simulink model "RflysimIndoorController_r2018b"  (R2018b)
settings: Solver=ode4  StartTime=0.0  StopTime=inf  FixedStep=ts  MaxStep=0.6  RelTol=1e-3
values from neighbouring files (symbols this model uses):
  l_v = 5    [RflyMain.m]    (also in RflyMain_N12_V6.m; RflyMain_N6_V3.m; RflyMain_N6_V4.m; RflyMain_V2.m)
  p_left_encircle = zeros(length(p_radius(:,1)),2)    [RflyMain.m]
  p_radius = [curve_x;curve_y]'    [RflyMain.m]
  p_right_encircle = zeros(length(p_radius(:,1)),2)    [RflyMain.m]
  p_target = [200,10]    [RflyMain.m]    (also in RflyMain_N12_V6.m; RflyMain_N6_V3.m; RflyMain_N6_V4.m; RflyMain_V2.m)
  ra = 0.6    [RflyMain.m]    (also in RflyMain_N12_V6.m; RflyMain_N6_V3.m; RflyMain_N6_V4.m; RflyMain_V2.m)
  rs = 0.25    [RflyMain.m]    (also in RflyMain_N12_V6.m; RflyMain_N6_V3.m; RflyMain_N6_V4.m; RflyMain_V2.m)
  tunnel_left = [90,20;147,14]    [RflyMain.m]
  tunnel_right = [90,1;147,7]    [RflyMain.m]
  v_max = 2    [RflyMain.m]    (also in RflyMain_N12_V6.m = 3; RflyMain_N6_V3.m = 3; RflyMain_N6_V4.m = 3; RflyMain_V2.m = 3)
undefined symbols (not defined in the file or in its folder): Twist
libraries: robotlib x7
settings Model: Creator=51078  LastModifiedBy=root
settings SFSimCC: SimUseLocalCustomCode=off
settings RTWCC: RTWUseLocalCustomCode=off
settings CodeAppCC: StateflowObjectComments=on

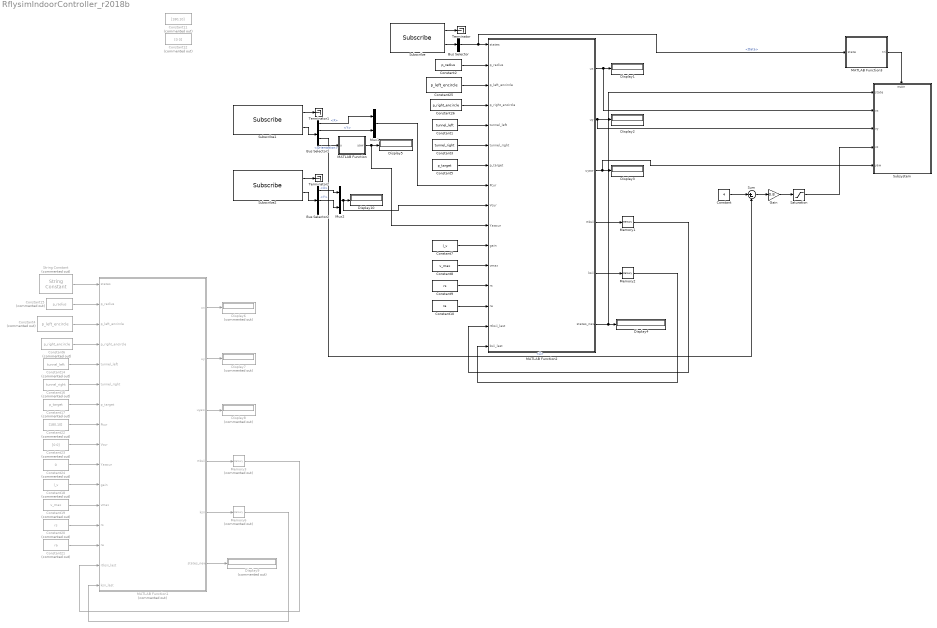
== system RflysimIndoorController_r2018b ==
  Bus Selector : BusSelector  OutputSignals=Data
  Bus Selector1 : BusSelector  OutputSignals=Pose.Position.X,Pose.Position.Y,Pose.Position.Z,Pose.Orientation
  Bus Selector2 : BusSelector  OutputSignals=Twist.Linear.X,Twist.Linear.Y,Twist.Linear.Z
  Constant : Constant  Value=4
  Constant1 : Constant  Value=tunnel_left
  Constant10 : Constant  Value=ra
  Constant11 : Constant  Commented=on  Value=[180,10]
  Constant12 : Constant  Commented=on  Value=[0 0]
  Constant14 : Constant  Commented=on  Value=tunnel_left
  Constant15 : Constant  Commented=on  Value=p_radius
  Constant16 : Constant  Commented=on  Value=tunnel_right
  Constant17 : Constant  Commented=on  Value=p_target
  Constant18 : Constant  Commented=on  Value=l_v
  Constant19 : Constant  Commented=on  Value=v_max
  Constant2 : Constant  Value=p_radius
  Constant20 : Constant  Commented=on  Value=rs
  Constant21 : Constant  Commented=on  Value=ra
  Constant22 : Constant  Commented=on  Value=[180,10]
  Constant23 : Constant  Commented=on  Value=[0 0]
  Constant24 : Constant  Commented=on  Value=0
  Constant25 : Constant  Value=p_left_encircle
  Constant26 : Constant  Value=p_right_encircle
  Constant3 : Constant  Value=tunnel_right
  Constant4 : Constant  Commented=on  Value=p_left_encircle
  Constant5 : Constant  Value=p_target
  Constant6 : Constant  Commented=on  Value=p_right_encircle
  Constant7 : Constant  Value=l_v
  Constant8 : Constant  Value=v_max
  Constant9 : Constant  Value=rs
  Display{1..5,10} (6 alike) : Display
  Display{6..9} (4 alike) : Display  Commented=on
  Gain : Gain  Gain=0.8
  MATLAB Function : MATLAB Function  TreatAsAtomicUnit=on
  MATLAB Function1 : MATLAB Function  Commented=on  TreatAsAtomicUnit=on
  MATLAB Function2 : MATLAB Function  TreatAsAtomicUnit=on
  MATLAB Function3 : MATLAB Function  TreatAsAtomicUnit=on
  Memory1 : Memory
  Memory2 : Memory
  Memory3 : Memory  Commented=on
  Memory6 : Memory  Commented=on
  Mux1 : Mux  Inputs=2
  Mux2 : Mux  Inputs=2
  Saturation : Saturate  UpperLimit=2  LowerLimit=-2
  String Constant : StringConstant  Commented=on  String="\"task_pass_through\""
  Subscribe : robotlib/Subscribe  topicSource=Select from ROS network  topic=/drone_1/state  messageType=std_msgs/UInt64  sampleTime=-1  messageQueueLength=1
  Subscribe1 : robotlib/Subscribe  topicSource=Select from ROS network  topic=/mavros/local_position/pose  messageType=geometry_msgs/PoseStamped  sampleTime=-1  messageQueueLength=1
  Subscribe2 : robotlib/Subscribe  topicSource=Select from ROS network  topic=/mavros/local_position/velocity_local  messageType=geometry_msgs/TwistStamped  sampleTime=-1  messageQueueLength=1
  Subsystem : Subsystem
  Sum : Sum  Inputs=|+-
  Terminator : Terminator
  Terminator1 : Terminator
  Terminator2 : Terminator
  wires:
  Subscribe1/1 -> Terminator1/1
  Subscribe1/2 -> Bus Selector1/1
  Constant15/1 -> MATLAB Function1/2(p_radius)
  Constant4/1 -> MATLAB Function1/3(p_left_encircle)
  Constant6/1 -> MATLAB Function1/4(p_right_encircle)
  Constant14/1 -> MATLAB Function1/5(tunnel_left)
  Constant16/1 -> MATLAB Function1/6(tunnel_right)
  Constant17/1 -> MATLAB Function1/7(p_target)
  Bus Selector1/2 -> Mux1/2  "<Y>"
  Constant18/1 -> MATLAB Function1/11(gain)
  Constant19/1 -> MATLAB Function1/12(vmax)
  Constant20/1 -> MATLAB Function1/13(rs)
  Constant21/1 -> MATLAB Function1/14(ra)
  MATLAB Function1/4(rtksii) -> Memory3/1
  Memory3/1 -> MATLAB Function1/15(rtksii_last)
  MATLAB Function1/5(ksii) -> Memory6/1
  Memory6/1 -> MATLAB Function1/16(ksii_last)
  String Constant/1 -> MATLAB Function1/1(states)
  Constant22/1 -> MATLAB Function1/8(Pcur)
  Constant23/1 -> MATLAB Function1/9(Vcur)
  Constant24/1 -> MATLAB Function1/10(Yawcur)
  MATLAB Function1/1(ux) -> Display6/1
  MATLAB Function1/2(uy) -> Display7/1
  MATLAB Function1/3(uyaw) -> Display8/1
  MATLAB Function1/6(states_new) -> Display9/1
  MATLAB Function2/4(rtksii) -> Memory1/1
  Constant9/1 -> MATLAB Function2/13(rs)
  Constant2/1 -> MATLAB Function2/2(p_radius)
  MATLAB Function2/3(uyaw) -> Subsystem/5(yaw), Display3/1
  Constant5/1 -> MATLAB Function2/7(p_target)
  Constant7/1 -> MATLAB Function2/11(gain)
  Constant25/1 -> MATLAB Function2/3(p_left_encircle)
  Memory1/1 -> MATLAB Function2/15(rtksii_last)
  Constant10/1 -> MATLAB Function2/14(ra)
  Constant26/1 -> MATLAB Function2/4(p_right_encircle)
  Mux2/1 -> MATLAB Function2/9(Vcur), Display10/1
  Constant1/1 -> MATLAB Function2/5(tunnel_left)
  Memory2/1 -> MATLAB Function2/16(ksii_last)
  Constant3/1 -> MATLAB Function2/6(tunnel_right)
  Mux1/1 -> MATLAB Function2/8(Pcur)
  MATLAB Function2/1(ux) -> Subsystem/2(vx), Display1/1
  MATLAB Function/1(yaw) -> MATLAB Function2/10(Yawcur), Display5/1
  MATLAB Function2/5(ksii) -> Memory2/1
  Constant8/1 -> MATLAB Function2/12(vmax)
  Subscribe/1 -> Terminator/1
  Subscribe/2 -> Bus Selector/1
  Bus Selector/1 -> MATLAB Function3/1(state), MATLAB Function2/1(states)  "<Data>"
  Bus Selector2/2 -> Mux2/2  "<Y>"
  Bus Selector2/1 -> Mux2/1  "<X>"
  Subscribe2/2 -> Bus Selector2/1
  Subscribe2/1 -> Terminator2/1
  Bus Selector1/4 -> MATLAB Function/1(u)  "<Orientation>"
  MATLAB Function3/1(tri) -> Subsystem/Enable
  MATLAB Function2/6(states_new) -> Subsystem/1(state), Display4/1
  MATLAB Function2/2(uy) -> Subsystem/3(vy), Display2/1
  Bus Selector1/1 -> Mux1/1  "<X>"
  Constant/1 -> Sum/1
  Bus Selector1/3 -> Sum/2  "<Z>"
  Sum/1 -> Gain/1
  Gain/1 -> Saturation/1
  Saturation/1 -> Subsystem/4(vz)

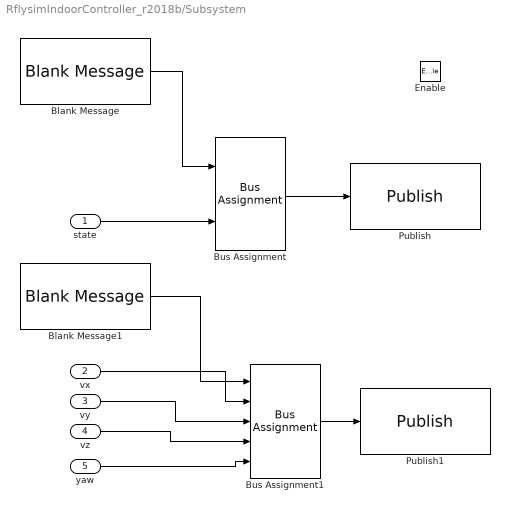
== system RflysimIndoorController_r2018b/Subsystem ==
  state : Inport
  vx : Inport  Port=2
  vy : Inport  Port=3
  vz : Inport  Port=4
  yaw : Inport  Port=5
  Enable : EnablePort
  Blank Message : robotlib/Blank Message  messageClass=Message  entityType=std_msgs/UInt64  messageType=std_msgs/UInt64  SampleTime=inf
      settings: SourceProductBaseCode=RO
  Blank Message1 : robotlib/Blank Message  messageClass=Message  entityType=geometry_msgs/TwistStamped  messageType=geometry_msgs/TwistStamped  SampleTime=inf
      settings: SourceProductBaseCode=RO
  Bus Assignment : BusAssignment  AssignedSignals=Data
  Bus Assignment1 : BusAssignment  AssignedSignals=Twist.Linear.X,Twist.Linear.Y,Twist.Linear.Z,Twist.Angular.Z
  Publish : robotlib/Publish  topicSource=Specify your own  topic=/drone_1/state  messageType=std_msgs/UInt64  messageQueueLength=1
      settings: SourceProductBaseCode=RO
  Publish1 : robotlib/Publish  topicSource=Select from ROS network  topic=/mavros/setpoint_velocity/cmd_vel  messageType=geometry_msgs/TwistStamped  messageQueueLength=1
      settings: SourceProductBaseCode=RO
  wires:
  Blank Message/1 -> Bus Assignment/1
  state/1 -> Bus Assignment/2
  Bus Assignment/1 -> Publish/1
  Bus Assignment1/1 -> Publish1/1
  Blank Message1/1 -> Bus Assignment1/1
  vx/1 -> Bus Assignment1/2
  vy/1 -> Bus Assignment1/3
  yaw/1 -> Bus Assignment1/5
  vz/1 -> Bus Assignment1/4

== matlab function RflysimIndoorController_r2018b/MATLAB Function1 ==
  data: states input; p_radius input; p_left_encircle input; p_right_encircle input; tunnel_left input; ux output; uy output; tunnel_right input; p_target input; Pcur input; Vcur input; Yawcur input; gain input; vmax input; uyaw output; rtksii output size=[N,1]; ksii output size=[N,2]; rs input; ra input; rtksii_last input; ksii_last input; states_new output
function [ux,uy,uyaw,rtksii,ksii,states_new]  = mytunnel(states,p_radius,p_left_encircle,p_right_encircle,tunnel_left,tunnel_right,p_target,Pcur,Vcur,Yawcur,gain,vmax,rs,ra,rtksii_last,ksii_last)
Pcur=Pcur';
Vcur=Vcur';
p_target=p_target';

N=1;
[u_encircle,ux_encircle,uy_encircle,uyaw_encircle,leader_locate,rtksii,ksii,dist_encircle]  = Encirclement(p_radius,p_left_encircle,p_right_encircle,p_target,Pcur,Vcur,Yawcur,gain,vmax,rs,ra,rtksii_last,ksii_last);
[u_pass,ux_pass,uy_pass,tunnel_locate,bottem_tunnel_locate,dist_tunnel]  = TixingTunnel(tunnel_left,tunnel_right,Pcur,Vcur,N,gain,vmax,rs,ra);

ux=zeros(N,1);
uy=zeros(N,1);
uyaw=zeros(N,1);
states_new="";
if states=="task_out_search"
    ux=ux_encircle;
    uy=uy_encircle;
    uyaw=uyaw_encircle;
    if tunnel_locate~=1
        states_new="task_out_search";
    elseif tunnel_locate==1
        states_new="task_pass_through";
    end
end

if states=="task_pass_through"
    ux=ux_pass;
    uy=uy_pass;
    uyaw=zeros(N,1);
    if tunnel_locate==1
        states_new="task_pass_through";
    elseif tunnel_locate~=1
        states_new="task_in_search";
    end
end

== matlab function RflysimIndoorController_r2018b/MATLAB Function2 ==
  data: states input; p_radius input; p_left_encircle input; p_right_encircle input; tunnel_left input; ux output; uy output; tunnel_right input; p_target input; Pcur input; Vcur input; Yawcur input; gain input; vmax input; uyaw output; rtksii output size=[N,1]; ksii output size=[N,2]; rs input; ra input; rtksii_last input; ksii_last input; states_new output
function [ux,uy,uyaw,rtksii,ksii,states_new]  = mytunnel(states,p_radius,p_left_encircle,p_right_encircle,tunnel_left,tunnel_right,p_target,Pcur,Vcur,Yawcur,gain,vmax,rs,ra,rtksii_last,ksii_last)
Pcur=Pcur';
Vcur=Vcur';
p_target=p_target';

N=1;
[u_encircle,ux_encircle,uy_encircle,uyaw_encircle,leader_locate,rtksii,ksii,dist_encircle]  = Encirclement(p_radius,p_left_encircle,p_right_encircle,p_target,Pcur,Vcur,Yawcur,gain,vmax,rs,ra,rtksii_last,ksii_last);
[u_pass,ux_pass,uy_pass,tunnel_locate,bottem_tunnel_locate,dist_tunnel]  = TixingTunnel(tunnel_left,tunnel_right,Pcur,Vcur,N,gain,vmax,rs,ra);

ux=zeros(N,1);
uy=zeros(N,1);
uyaw=zeros(N,1);
states_new=0;
if states==20
    ux=ux_encircle;
    uy=uy_encircle;
    uyaw=uyaw_encircle;
    if tunnel_locate~=1
        states_new=20;
    elseif tunnel_locate==1
        states_new=40;
    end
end

if states==40
    ux=ux_pass;
    uy=uy_pass;
    uyaw=zeros(N,1);
    if tunnel_locate==1
        states_new=40;
    elseif tunnel_locate~=1
        states_new=50;
    end
end

== matlab function RflysimIndoorController_r2018b/MATLAB Function ==
  data: u input; yaw output
function yaw = fcn(u)
q0=u.W;
q1=u.X;
q2=u.Y;
q3=u.Z;
yaw = atan2(2*(q0*q3+q1*q2), 1-2*(q2*q2+q3*q3));

== matlab function RflysimIndoorController_r2018b/MATLAB Function3 ==
  data: state input; tri output
function tri = fcn(state)
tri=0;
if state==20 || state==30 || state==40 
    tri=1;
end
